simulink model "demo_exakt_mimo"  (Simulink 2.20)
settings: Solver=ode45  StartTime=0.0  StopTime=5.0  MaxStep=0.1  RelTol=1e-3  AbsTol=1e-6
values from neighbouring files (symbols this model uses):
  x1 = x(j)    [fazrov_auton2.m]
  x2 = x(j+1)    [fazrov_auton2.m]    (also in fazrov_typ1.m = get_param(get_param(gcbh,'Parent'),'UserData'))
undefined symbols (not defined in the file or in its folder): v1, v2, x3, z1
libraries: NelinSys x4
CloseFcn:
  | ;slview('closediagram',bdroot);
settings Model: ConsistencyChecking=off  RTWPlaceOutputsASAP=off

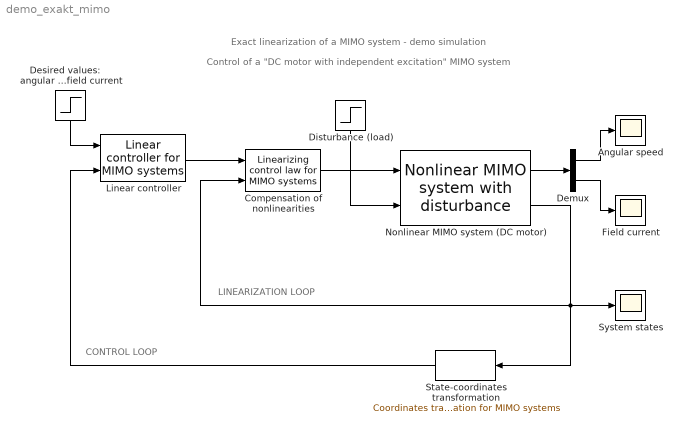
== system demo_exakt_mimo ==
  note: LINEARIZATION LOOP
  note: CONTROL LOOP
  note: Exact linearization of a MIMO system - demo simulation
  note: Control of a "DC motor with independent excitation" MIMO system
  " Desired values:     angular speed & field current" : Step  Orientation=down  Time=[0.3 4]  Before=[0 0.26]  After=[10 0.2]
  " Disturbance (load)" : Step  Orientation=down  Time=2  Before=0  After=0.2
  Angular speed : Scope
      settings: TickLabels=on  TimeRange=5  YMin=0  YMax=15  SaveToWorkspace=off  SaveName=ScopeData
  Compensation of nonlinearities : NelinSys/Nonlinear Systems Synthesis/Exact Linearization Blocks/Linearizing control law for MIMO systems  n=3  nout=2  vzorec=[1167173990052591/17592186044416000*x1*x3+1/40*x2+2/421245/x3*v1-1/2500*x2/x3*v2; 153846/9799*x3+10000/9799*v2]  vzorecP=0
  Demux : Demux  Outputs=2
  Field current : Scope
      settings: TickLabels=on  TimeRange=5  YMin=0  YMax=0.3  SaveToWorkspace=off  SaveName=ScopeData
  Linear controller : NelinSys/Nonlinear Systems Synthesis/Exact Linearization Blocks/Linear controller for MIMO systems  r=[2 1]  nout=2  kor=[-20 -20 -60 -20 -60]  integ=on
  Nonlinear MIMO system (DC motor) : NelinSys/Nonlinear Systems Synthesis/Nonlinear MIMO system with disturbance  n=3  F=[84.249*x2*x3; -165.8654*x1*x3-62.5*x2; -15.3846*x3]  Fp=0  G=[0 0; 2500 0; 0 0.9799]  Gp=0  H=[x1; x3]  Hp=0  E=[-31.746*z1; 0; 0]  Ep=0  pp=[0; 0; 1e-9]
  State-coordinates transformation : NelinSys/Nonlinear Systems Synthesis/Exact Linearization Blocks/Coordinates transformation for MIMO systems  Orientation=left  n=3  r=[2 1]  Z=[x1; 84.249*x2*x3; x3]  Zp=0
  System states : Scope
      settings: TickLabels=on  TimeRange=5  YMin=0  YMax=15  SaveToWorkspace=off  SaveName=ScopeData
  wires:
  Linear controller/1 -> Compensation of nonlinearities/1
  State-coordinates transformation/1 -> Linear controller/2
  " Desired values:     angular speed & field current"/1 -> Linear controller/1
  Nonlinear MIMO system (DC motor)/2 -> State-coordinates transformation/1, Compensation of nonlinearities/2, System states/1
  Compensation of nonlinearities/1 -> Nonlinear MIMO system (DC motor)/1
  " Disturbance (load)"/1 -> Nonlinear MIMO system (DC motor)/2
  Nonlinear MIMO system (DC motor)/1 -> Demux/1
  Demux/1 -> Angular speed/1
  Demux/2 -> Field current/1
